simulink library "DF3000_V2_Common"  (R2023b)
settings: Solver=VariableStepAuto  StartTime=0.0  StopTime=10.0  RelTol=1e-3
undefined symbols (not defined in the file): ArmDirSelected, Geom, Newton, Raphson
libraries: simulink_extras x14, $bdroot x7, matrix_library x5, sharedtransform x5, aerolibasang x3, aerolibtransform2 x1
settings Model: Creator=ZJRY  LastModifiedBy=qu_yx

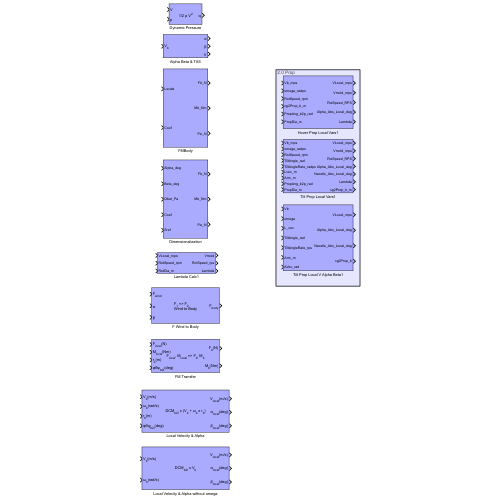
[thumbnail: Simulink's stored preview of the top-level diagram]
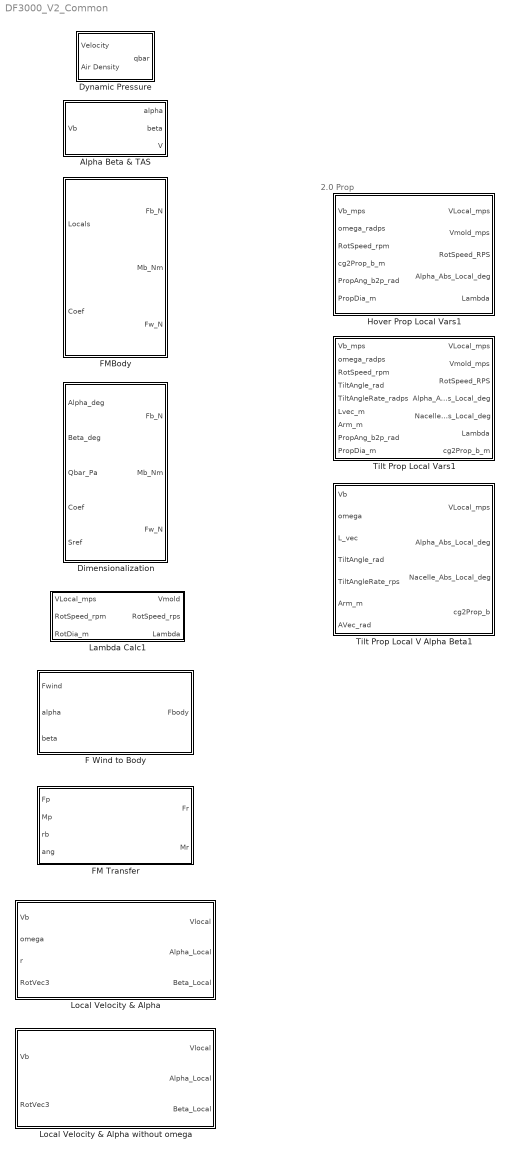
== system DF3000_V2_Common ==
  note: 2.0 Prop
  Alpha Beta & TAS : Subsystem
      mask Display:
      | port_label('input',1,'V_b','texmode','on');
      | port_label('output',1,'\alpha','texmode','on');
      | port_label('output',2,'\beta','texmode','on');
      | port_label('output',3,'V','texmode','on');
  Dimensionalization : Subsystem
  Dynamic Pressure : Subsystem
      mask Display:
      | disp('1/2 \rho V^2', 'texmode','on');
      | port_label('input',1,'V','texmode','on');
      | port_label('input',2,'\rho','texmode','on');
      | port_label('output',1,'q','texmode','on');
  F Wind to Body : Subsystem
      mask Display:
      | disp(['F_1 => F_2 \newline' ...
      |     'Wind to Body'], 'texmode','on');
      | port_label('input',1,'F_{wind}','texmode','on');
      | port_label('input',2,'\alpha','texmode','on');
      | port_label('input',3,'\beta','texmode','on');
      | port_label('output',1,'F_{body}','texmode','on');
  FM Transfer : Subsystem
      mask Display:
      | disp('F_{local}, M_{local} => F_b, M_b', 'texmode','on');
      | port_label('input',1,'F_{local}(N)','texmode','on');
      | port_label('input',2,'M_{local}(Nm)','texmode','on');
      | port_label('input',3,'r_b(m)','texmode','on');
      | port_label('input',4,'\phi\theta\psi_{b2l}(deg)','texmode','on');
      | port_label('output',1,'F_b(N)','texmode','on');
      | port_label('output',2,'M_b(Nm)','texmode','on');
  FMBody : Subsystem
  Hover Prop Local Vars1 : Subsystem
  Lambda Calc1 : Subsystem
  Local Velocity & Alpha : Subsystem
      mask Display:
      | disp('DCM_{b2l} x (V_b + \omega_b x r_b)', 'texmode','on');
      | port_label('input',1,'V_b(m/s)','texmode','on');
      | port_label('input',2,'\omega_b(rad/s)','texmode','on');
      | port_label('input',3,'r_b(m)','texmode','on');
      | port_label('input',4,'\phi\theta\psi_{b2l}(deg)','texmode','on');
      | port_label('output',1,'V_{local}(m/s)','texmode','on');
      | port_label('output',2,'\alpha_{local}(deg)','texmode','on');
      | port_label('output',3,'\beta_{local}(deg)','texmode','on');
  Local Velocity & Alpha without omega : Subsystem
      mask Display:
      | disp('DCM_{b2l} x V_b', 'texmode','on');
      | port_label('input',1,'V_b(m/s)','texmode','on');
      | port_label('input',2,'\omega_b(rad/s)','texmode','on');
      | port_label('output',1,'V_{local}(m/s)','texmode','on');
      | port_label('output',2,'\alpha_{local}(deg)','texmode','on');
      | port_label('output',3,'\beta_{local}(deg)','texmode','on');
  Tilt Prop Local V Alpha Beta1 : Subsystem
  Tilt Prop Local Vars1 : Subsystem

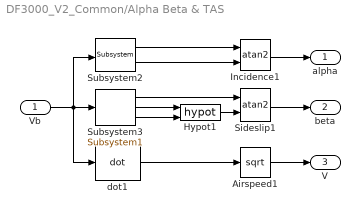
== system DF3000_V2_Common/Alpha Beta & TAS ==
  Vb : Inport
  Airspeed1 : Sqrt  AlgorithmType=Newton-Raphson
  Hypot1 : Math  Operator=hypot
  Incidence1 : Trigonometry  Operator=atan2
  Sideslip1 : Trigonometry  Operator=atan2
  Subsystem2 : aerolibasang/Incidence, Sideslip, & Airspeed/Subsystem  SystemSampleTime=-1  VariantActivationTime=update diagram  AllowFlexibleInterface=on  Latency=0  AutoFrameSizeCalculation=off
  Subsystem3 : aerolibasang/Incidence, Sideslip, & Airspeed/Subsystem1  SystemSampleTime=-1  VariantActivationTime=update diagram  AllowFlexibleInterface=on  Latency=0  AutoFrameSizeCalculation=off
  dot1 : aerolibasang/Incidence, Sideslip, & Airspeed/dot  SystemSampleTime=-1  VariantActivationTime=update diagram  AllowFlexibleInterface=on  Latency=0  AutoFrameSizeCalculation=off
  alpha : Outport
  beta : Outport  Port=2
  V : Outport  Port=3
  wires:
  Vb/1 -> Subsystem3/1, dot1/1, Subsystem2/1
  Subsystem2/2 -> Incidence1/2
  Subsystem3/2 -> Hypot1/1
  Subsystem2/1 -> Incidence1/1
  Subsystem3/3 -> Hypot1/2
  dot1/1 -> Airspeed1/1
  Subsystem3/1 -> Sideslip1/1
  Sideslip1/1 -> beta/1
  Hypot1/1 -> Sideslip1/2
  Airspeed1/1 -> V/1
  Incidence1/1 -> alpha/1

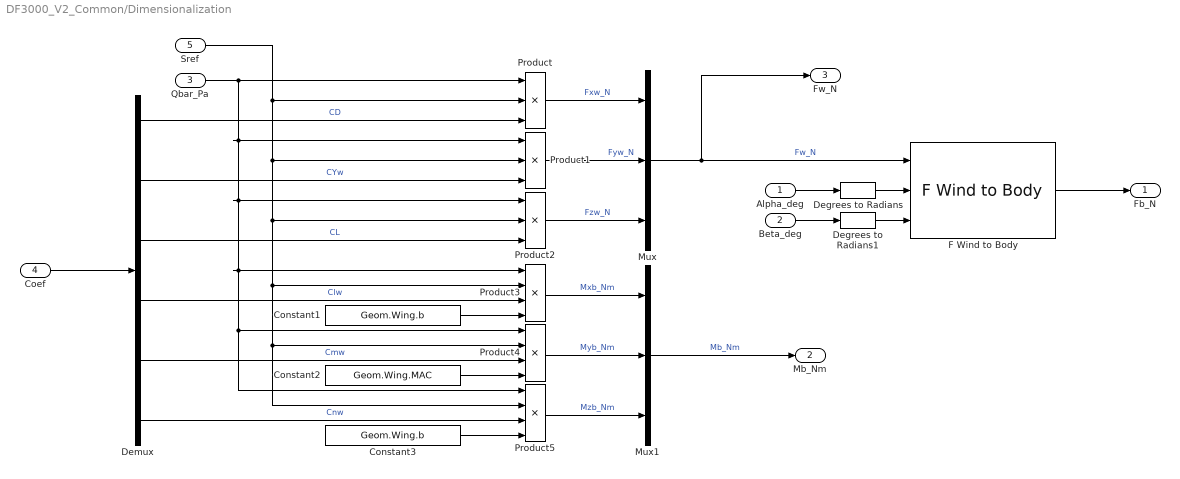
== system DF3000_V2_Common/Dimensionalization ==
  Alpha_deg : Inport
  Beta_deg : Inport  Port=2
  Qbar_Pa : Inport  Port=3
  Coef : Inport  Port=4
  Sref : Inport  Port=5
  Constant1 : Constant  Value=Geom.Wing.b
  Constant2 : Constant  Value=Geom.Wing.MAC
  Constant3 : Constant  Value=Geom.Wing.b
  Degrees to Radians : simulink_extras/Transformations/Degrees to Radians
  Degrees to Radians1 : simulink_extras/Transformations/Degrees to Radians
  Demux : Demux  Outputs=6
  F Wind to Body : $bdroot/F Wind to Body  SystemSampleTime=-1  VariantActivationTime=update diagram  AllowFlexibleInterface=on  Latency=0  AutoFrameSizeCalculation=off
  Mux : Mux  Inputs=3
  Mux1 : Mux  Inputs=3
  Product : Product  Inputs=3
  Product1 : Product  Inputs=3
  Product2 : Product  Inputs=3
  Product3 : Product  Inputs=4
  Product4 : Product  Inputs=4
  Product5 : Product  Inputs=4
  Fb_N : Outport
  Mb_Nm : Outport  Port=2
  Fw_N : Outport  Port=3
  wires:
  Beta_deg/1 -> Degrees to Radians1/1
  Alpha_deg/1 -> Degrees to Radians/1
  F Wind to Body/1 -> Fb_N/1
  Mux1/1 -> Mb_Nm/1  "Mb_Nm"
  Mux/1 -> F Wind to Body/1, Fw_N/1  "Fw_N"
  Constant1/1 -> Product3/4
  Constant3/1 -> Product5/4
  Constant2/1 -> Product4/4
  Sref/1 -> Product5/2, Product4/2, Product3/2, Product2/2, Product1/2, Product/2
  Demux/6 -> Product5/3  "Cnw"
  Demux/5 -> Product4/3  "Cmw"
  Demux/4 -> Product3/3  "Clw"
  Product3/1 -> Mux1/1  "Mxb_Nm"
  Product4/1 -> Mux1/2  "Myb_Nm"
  Product5/1 -> Mux1/3  "Mzb_Nm"
  Product2/1 -> Mux/3  "Fzw_N"
  Product1/1 -> Mux/2  "Fyw_N"
  Product/1 -> Mux/1  "Fxw_N"
  Qbar_Pa/1 -> Product1/1, Product2/1, Product4/1, Product5/1, Product3/1, Product/1
  Demux/3 -> Product2/3  "CL"
  Demux/2 -> Product1/3  "CYw"
  Demux/1 -> Product/3  "CD"
  Coef/1 -> Demux/1
  Degrees to Radians/1 -> F Wind to Body/2
  Degrees to Radians1/1 -> F Wind to Body/3

== system DF3000_V2_Common/Dynamic Pressure ==
  Velocity : Inport
  Air Density : Inport  Port=2
  1/2rhoV^2 : Gain  Gain=1/2  SaturateOnIntegerOverflow=on  OutDataTypeStr=Inherit: Same as input  ParamDataTypeStr=Inherit: Same as input
  Add : Sum  Inputs=+++
  Demux1 : Demux  Outputs=3
  Product2 : Product  InputSameDT=on  SaturateOnIntegerOverflow=on  OutDataTypeStr=Inherit: Same as first input
  Square : Math  Operator=square
  Square1 : Math  Operator=square
  Square2 : Math  Operator=square
  qbar : Outport  InitialOutput=0  VectorParamsAs1DForOutWhenUnconnected=off
  wires:
  Air Density/1 -> Product2/2
  Product2/1 -> 1/2rhoV^2/1
  1/2rhoV^2/1 -> qbar/1
  Add/1 -> Product2/1
  Demux1/3 -> Square/1
  Velocity/1 -> Demux1/1
  Square/1 -> Add/3
  Demux1/1 -> Square2/1
  Demux1/2 -> Square1/1
  Square1/1 -> Add/2
  Square2/1 -> Add/1

== system DF3000_V2_Common/F Wind to Body ==
  Fwind : Inport  PortDimensions=3
  alpha : Inport  Port=2
  beta : Inport  Port=3
  Direction Cosine Matrix Body to Wind : aerolibtransform2/Direction Cosine Matrix Body to Wind
  Matrix Multiply3 : Product  Multiplication=Matrix(*)
  Mux : Mux  Inputs=2
  Wind to Body : Math  Operator=transpose
  Fbody : Outport  PortDimensions=3
  wires:
  Matrix Multiply3/1 -> Fbody/1
  Direction Cosine Matrix Body to Wind/1 -> Wind to Body/1
  Fwind/1 -> Matrix Multiply3/2
  Mux/1 -> Direction Cosine Matrix Body to Wind/1
  alpha/1 -> Mux/1
  beta/1 -> Mux/2
  Wind to Body/1 -> Matrix Multiply3/1

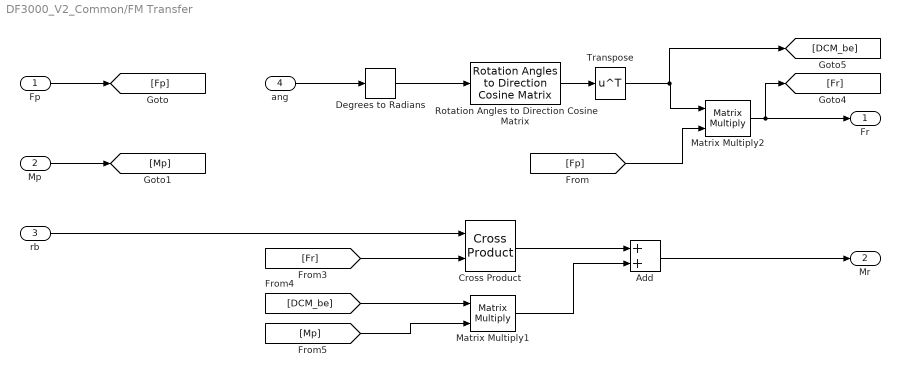
== system DF3000_V2_Common/FM Transfer ==
  Fp : Inport  PortDimensions=3
  Mp : Inport  Port=2  PortDimensions=3
  rb : Inport  Port=3  PortDimensions=3
  ang : Inport  Port=4  PortDimensions=3
  Add : Sum
  Cross Product : matrix_library/Cross Product
  Degrees to Radians : simulink_extras/Transformations/Degrees to Radians
  Matrix Multiply1 : Product  Multiplication=Matrix(*)
  Matrix Multiply2 : Product  Multiplication=Matrix(*)
  Rotation Angles to Direction Cosine Matrix : sharedtransform/Rotation Angles to Direction Cosine Matrix  rotationOrder=XYZ  aMode=aMode
  Transpose : Math  Operator=transpose
  Fr : Outport  PortDimensions=3
  Mr : Outport  Port=2  PortDimensions=3
  wires:
  rb/1 -> Cross Product/1
  [Fp] -> Matrix Multiply2/2
  Rotation Angles to Direction Cosine Matrix/1 -> Transpose/1
  Degrees to Radians/1 -> Rotation Angles to Direction Cosine Matrix/1
  Fp/1 -> [Fp]
  Transpose/1 -> Matrix Multiply2/1, [DCM_be]
  Mp/1 -> [Mp]
  Add/1 -> Mr/1
  ang/1 -> Degrees to Radians/1
  Matrix Multiply2/1 -> Fr/1, [Fr]
  [DCM_be] -> Matrix Multiply1/1
  [Fr] -> Cross Product/2
  Cross Product/1 -> Add/1
  [Mp] -> Matrix Multiply1/2
  Matrix Multiply1/1 -> Add/2

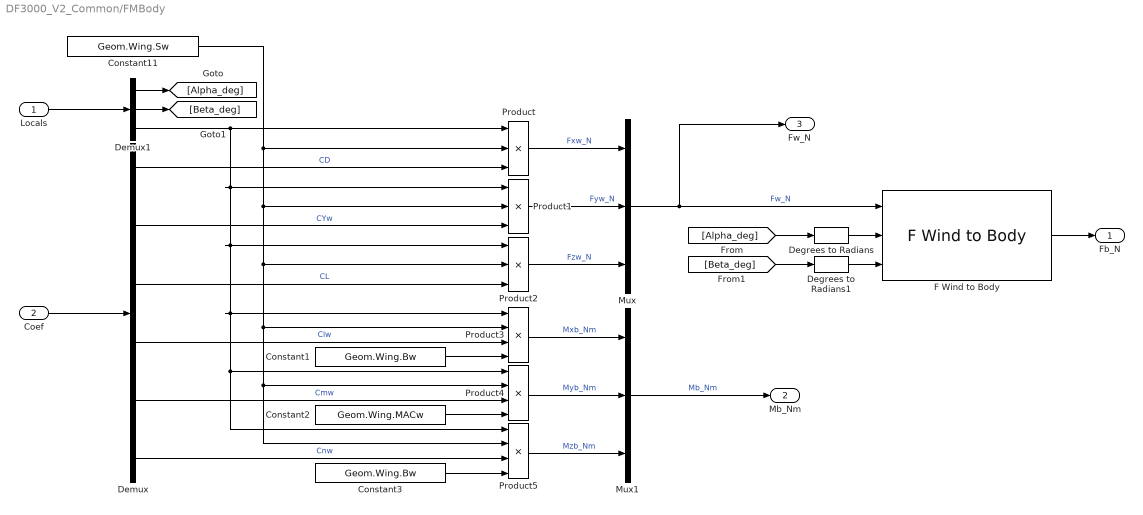
== system DF3000_V2_Common/FMBody ==
  Locals : Inport
  Coef : Inport  Port=2
  Constant1 : Constant  Value=Geom.Wing.Bw
  Constant11 : Constant  Value=Geom.Wing.Sw
  Constant2 : Constant  Value=Geom.Wing.MACw
  Constant3 : Constant  Value=Geom.Wing.Bw
  Degrees to Radians : simulink_extras/Transformations/Degrees to Radians
  Degrees to Radians1 : simulink_extras/Transformations/Degrees to Radians
  Demux : Demux  Outputs=6
  Demux1 : Demux  Outputs=3
  F Wind to Body : $bdroot/F Wind to Body  SystemSampleTime=-1  VariantActivationTime=update diagram  AllowFlexibleInterface=on  Latency=0  AutoFrameSizeCalculation=off
  Mux : Mux  Inputs=3
  Mux1 : Mux  Inputs=3
  Product : Product  Inputs=3
  Product1 : Product  Inputs=3
  Product2 : Product  Inputs=3
  Product3 : Product  Inputs=4
  Product4 : Product  Inputs=4
  Product5 : Product  Inputs=4
  Fb_N : Outport
  Mb_Nm : Outport  Port=2
  Fw_N : Outport  Port=3
  wires:
  [Beta_deg] -> Degrees to Radians1/1
  [Alpha_deg] -> Degrees to Radians/1
  Demux1/1 -> [Alpha_deg]
  F Wind to Body/1 -> Fb_N/1
  Mux1/1 -> Mb_Nm/1  "Mb_Nm"
  Mux/1 -> F Wind to Body/1, Fw_N/1  "Fw_N"
  Constant1/1 -> Product3/4
  Constant3/1 -> Product5/4
  Constant2/1 -> Product4/4
  Constant11/1 -> Product5/2, Product4/2, Product3/2, Product2/2, Product1/2, Product/2
  Demux/6 -> Product5/3  "Cnw"
  Demux/5 -> Product4/3  "Cmw"
  Demux/4 -> Product3/3  "Clw"
  Product3/1 -> Mux1/1  "Mxb_Nm"
  Product4/1 -> Mux1/2  "Myb_Nm"
  Product5/1 -> Mux1/3  "Mzb_Nm"
  Product2/1 -> Mux/3  "Fzw_N"
  Product1/1 -> Mux/2  "Fyw_N"
  Product/1 -> Mux/1  "Fxw_N"
  Demux1/3 -> Product1/1, Product2/1, Product4/1, Product5/1, Product3/1, Product/1
  Locals/1 -> Demux1/1
  Demux/3 -> Product2/3  "CL"
  Demux/2 -> Product1/3  "CYw"
  Demux/1 -> Product/3  "CD"
  Coef/1 -> Demux/1
  Degrees to Radians/1 -> F Wind to Body/2
  Degrees to Radians1/1 -> F Wind to Body/3
  Demux1/2 -> [Beta_deg]

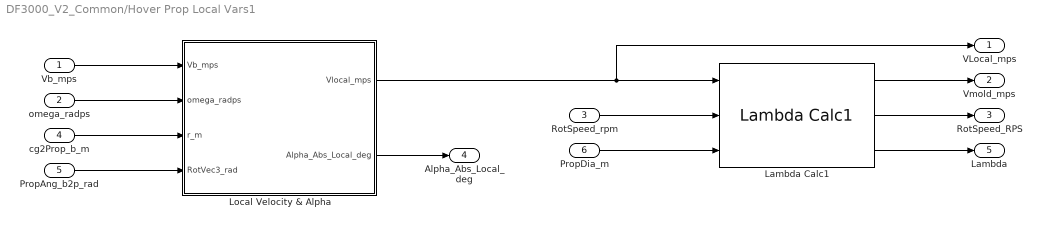
== system DF3000_V2_Common/Hover Prop Local Vars1 ==
  Vb_mps : Inport
  omega_radps : Inport  Port=2
  RotSpeed_rpm : Inport  Port=3
  cg2Prop_b_m : Inport  Port=4
  PropAng_b2p_rad : Inport  Port=5
  PropDia_m : Inport  Port=6
  Lambda Calc1 : $bdroot/Lambda Calc1  SystemSampleTime=-1  VariantActivationTime=update diagram  AllowFlexibleInterface=on  Latency=0  AutoFrameSizeCalculation=off
  Local Velocity & Alpha : Subsystem
  VLocal_mps : Outport
  Vmold_mps : Outport  Port=2
  RotSpeed_RPS : Outport  Port=3
  Alpha_Abs_Local_deg : Outport  Port=4
  Lambda : Outport  Port=5
  wires:
  omega_radps/1 -> Local Velocity & Alpha/2(omega_radps)
  RotSpeed_rpm/1 -> Lambda Calc1/2
  Local Velocity & Alpha/1(Vlocal_mps) -> Lambda Calc1/1, VLocal_mps/1
  Vb_mps/1 -> Local Velocity & Alpha/1(Vb_mps)
  Local Velocity & Alpha/2(Alpha_Abs_Local_deg) -> Alpha_Abs_Local_deg/1
  PropAng_b2p_rad/1 -> Local Velocity & Alpha/4(RotVec3_rad)
  cg2Prop_b_m/1 -> Local Velocity & Alpha/3(r_m)
  PropDia_m/1 -> Lambda Calc1/3
  Lambda Calc1/3 -> Lambda/1
  Lambda Calc1/2 -> RotSpeed_RPS/1
  Lambda Calc1/1 -> Vmold_mps/1

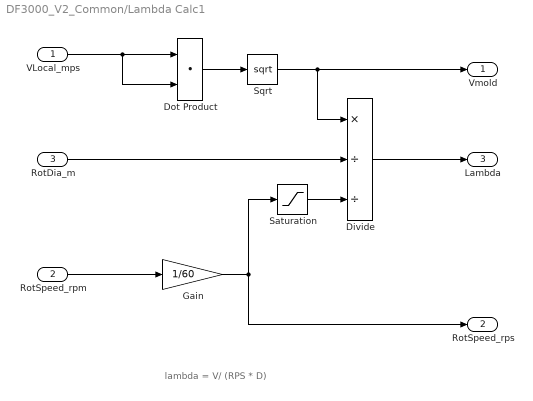
== system DF3000_V2_Common/Lambda Calc1 ==
  note: lambda = V/ (RPS * D)
  VLocal_mps : Inport
  RotSpeed_rpm : Inport  Port=2
  RotDia_m : Inport  Port=3
  Divide : Product  Inputs=*//
  Dot Product : DotProduct  OutDataTypeStr=Inherit: Inherit via internal rule
  Gain : Gain  Gain=1/60
  Saturation : Saturate  UpperLimit=10000  LowerLimit=0.0001
  Sqrt : Sqrt
  Vmold : Outport
  RotSpeed_rps : Outport  Port=2
  Lambda : Outport  Port=3
  wires:
  RotSpeed_rpm/1 -> Gain/1
  Gain/1 -> Saturation/1, RotSpeed_rps/1
  RotDia_m/1 -> Divide/2
  Divide/1 -> Lambda/1
  VLocal_mps/1 -> Dot Product/2, Dot Product/1
  Dot Product/1 -> Sqrt/1
  Saturation/1 -> Divide/3
  Sqrt/1 -> Vmold/1, Divide/1

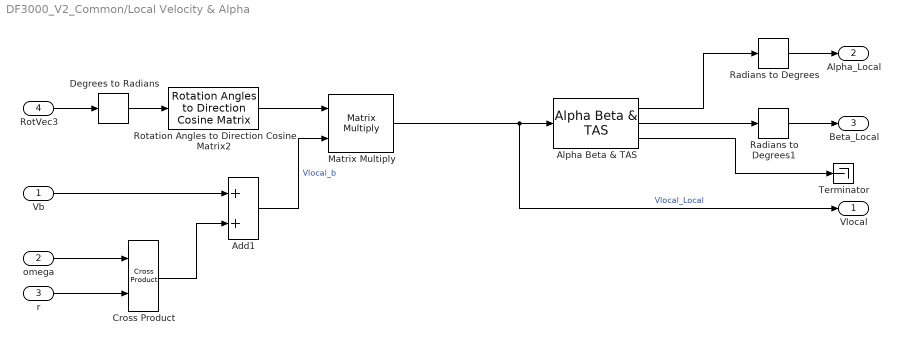
== system DF3000_V2_Common/Local Velocity & Alpha ==
  Vb : Inport
  omega : Inport  Port=2
  r : Inport  Port=3
  RotVec3 : Inport  Port=4
  Add1 : Sum
  Alpha Beta & TAS : $bdroot/Alpha Beta & TAS  SystemSampleTime=-1  VariantActivationTime=update diagram  AllowFlexibleInterface=on  Latency=0  AutoFrameSizeCalculation=off
  Cross Product : matrix_library/Cross Product
  Degrees to Radians : simulink_extras/Transformations/Degrees to Radians
  Matrix Multiply : Product  Multiplication=Matrix(*)
  Radians to Degrees : simulink_extras/Transformations/Radians to Degrees
  Radians to Degrees1 : simulink_extras/Transformations/Radians to Degrees
  Rotation Angles to Direction Cosine Matrix2 : sharedtransform/Rotation Angles to Direction Cosine Matrix  rotationOrder=XYZ  aMode=aMode
  Terminator : Terminator
  Vlocal : Outport
  Alpha_Local : Outport  Port=2
  Beta_Local : Outport  Port=3
  wires:
  Vb/1 -> Add1/1
  Add1/1 -> Matrix Multiply/2  "Vlocal_b"
  Cross Product/1 -> Add1/2
  r/1 -> Cross Product/2
  omega/1 -> Cross Product/1
  Matrix Multiply/1 -> Vlocal/1, Alpha Beta & TAS/1  "Vlocal_Local"
  Rotation Angles to Direction Cosine Matrix2/1 -> Matrix Multiply/1
  RotVec3/1 -> Degrees to Radians/1
  Alpha Beta & TAS/3 -> Terminator/1
  Degrees to Radians/1 -> Rotation Angles to Direction Cosine Matrix2/1
  Alpha Beta & TAS/1 -> Radians to Degrees/1
  Alpha Beta & TAS/2 -> Radians to Degrees1/1
  Radians to Degrees/1 -> Alpha_Local/1
  Radians to Degrees1/1 -> Beta_Local/1

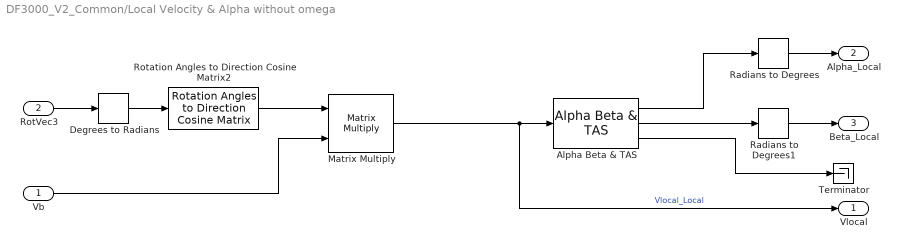
== system DF3000_V2_Common/Local Velocity & Alpha without omega ==
  Vb : Inport
  RotVec3 : Inport  Port=2
  Alpha Beta & TAS : $bdroot/Alpha Beta & TAS  SystemSampleTime=-1  VariantActivationTime=update diagram  AllowFlexibleInterface=on  Latency=0  AutoFrameSizeCalculation=off
  Degrees to Radians : simulink_extras/Transformations/Degrees to Radians
  Matrix Multiply : Product  Multiplication=Matrix(*)
  Radians to Degrees : simulink_extras/Transformations/Radians to Degrees
  Radians to Degrees1 : simulink_extras/Transformations/Radians to Degrees
  Rotation Angles to Direction Cosine Matrix2 : sharedtransform/Rotation Angles to Direction Cosine Matrix  rotationOrder=XYZ  aMode=aMode
  Terminator : Terminator
  Vlocal : Outport
  Alpha_Local : Outport  Port=2
  Beta_Local : Outport  Port=3
  wires:
  Radians to Degrees1/1 -> Beta_Local/1
  Radians to Degrees/1 -> Alpha_Local/1
  Alpha Beta & TAS/2 -> Radians to Degrees1/1
  Alpha Beta & TAS/1 -> Radians to Degrees/1
  Degrees to Radians/1 -> Rotation Angles to Direction Cosine Matrix2/1
  Alpha Beta & TAS/3 -> Terminator/1
  RotVec3/1 -> Degrees to Radians/1
  Rotation Angles to Direction Cosine Matrix2/1 -> Matrix Multiply/1
  Matrix Multiply/1 -> Alpha Beta & TAS/1, Vlocal/1  "Vlocal_Local"
  Vb/1 -> Matrix Multiply/2

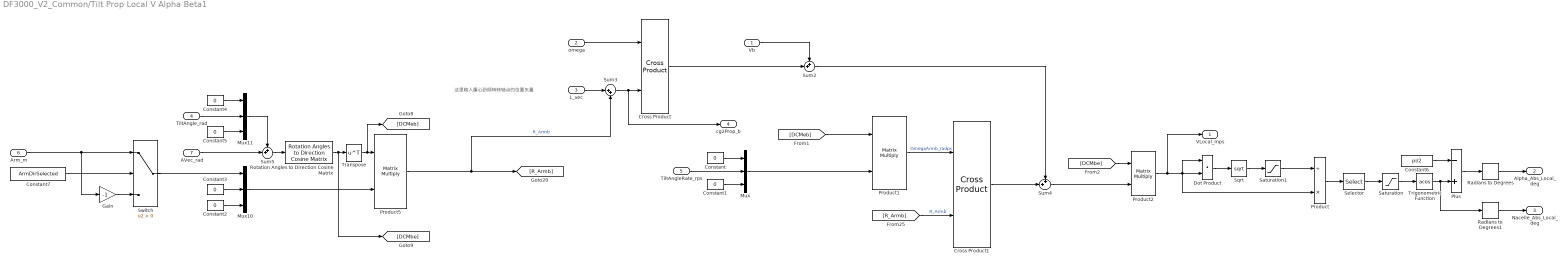
== system DF3000_V2_Common/Tilt Prop Local V Alpha Beta1 ==
  note: 这里输入重心到倾转转轴点的位置矢量
  Vb : Inport
  omega : Inport  Port=2
  L_vec : Inport  Port=3
  TiltAngle_rad : Inport  Port=4
  TiltAngleRate_rps : Inport  Port=5
  Arm_m : Inport  Port=6
  AVec_rad : Inport  Port=7
  Constant{,1..5} (6 alike) : Constant  Value=0
  Constant6 : Constant  Value=pi/2
  Constant7 : Constant  Value=ArmDirSelected
  Cross Product : matrix_library/Cross Product
  Cross Product1 : matrix_library/Cross Product
  Dot Product : DotProduct  OutDataTypeStr=Inherit: Inherit via internal rule
  Gain : Gain  Gain=-1
  Mux : Mux  Inputs=3
  Mux10 : Mux  Inputs=3
  Mux11 : Mux  Inputs=3
  Plus : Sum  Inputs=-+
  Product : Product  Inputs=/*
  Product1 : Product  Multiplication=Matrix(*)  InputSameDT=on  SaturateOnIntegerOverflow=on  OutDataTypeStr=Inherit: Same as first input
  Product2 : Product  Multiplication=Matrix(*)  InputSameDT=on  SaturateOnIntegerOverflow=on  OutDataTypeStr=Inherit: Same as first input
  Product5 : Product  Multiplication=Matrix(*)  InputSameDT=on  SaturateOnIntegerOverflow=on  OutDataTypeStr=Inherit: Same as first input
  Radians to Degrees : simulink_extras/Transformations/Radians to Degrees
  Radians to Degrees1 : simulink_extras/Transformations/Radians to Degrees
  Rotation Angles to Direction Cosine Matrix : sharedtransform/Rotation Angles to Direction Cosine Matrix  rotationOrder=XYZ  aMode=aMode
  Saturation : Saturate  UpperLimit=1  LowerLimit=-1
  Saturation1 : Saturate  UpperLimit=inf  LowerLimit=0.0001
  Selector : Selector  InputPortWidth=3  IndexOptions=Index vector (dialog)  Indices=[1]  OutputSizes=1
  Sqrt : Sqrt
  Sum2 : Sum  Inputs=++|
  Sum3 : Sum  Inputs=|++
  Sum4 : Sum  Inputs=++|
  Sum5 : Sum  Inputs=++|
  Switch : Switch  Criteria=u2 > Threshold  SaturateOnIntegerOverflow=off  InputSameDT=off
  Transpose : Math  Operator=transpose
  Trigonometric Function : Trigonometry  Operator=acos
  VLocal_mps : Outport
  Alpha_Abs_Local_deg : Outport  Port=2
  Nacelle_Abs_Local_deg : Outport  Port=3
  cg2Prop_b : Outport  Port=4
  wires:
  Constant5/1 -> Mux11/3
  Cross Product1/1 -> Sum4/2
  [R_Armb] -> Cross Product1/2  "R_Armb"
  TiltAngleRate_rps/1 -> Mux/2
  Product1/1 -> Cross Product1/1  "OmegaArmb_radps"
  [DCMeb] -> Product1/1
  Transpose/1 -> [DCMeb], Product5/1
  [DCMbe] -> Product2/1
  Sum3/1 -> cg2Prop_b/1, Cross Product/2
  Constant/1 -> Mux/1
  Product5/1 -> [R_Armb], Sum3/2  "R_Armb"
  Constant1/1 -> Mux/3
  Rotation Angles to Direction Cosine Matrix/1 -> [DCMbe], Transpose/1
  omega/1 -> Cross Product/1
  TiltAngle_rad/1 -> Mux11/2
  Cross Product/1 -> Sum2/2
  Mux10/1 -> Product5/2
  Sum2/1 -> Sum4/1
  AVec_rad/1 -> Sum5/2
  Sum4/1 -> Product2/2
  Sum5/1 -> Rotation Angles to Direction Cosine Matrix/1
  Constant4/1 -> Mux11/1
  Mux11/1 -> Sum5/1
  Mux/1 -> Product1/2
  Constant3/1 -> Mux10/2
  Constant2/1 -> Mux10/3
  Arm_m/1 -> Switch/1, Gain/1
  Gain/1 -> Switch/3
  Constant7/1 -> Switch/2
  Switch/1 -> Mux10/1
  Constant6/1 -> Plus/1
  Selector/1 -> Saturation/1
  Trigonometric Function/1 -> Radians to Degrees1/1, Plus/2
  Product/1 -> Selector/1
  Plus/1 -> Radians to Degrees/1
  Radians to Degrees/1 -> Alpha_Abs_Local_deg/1
  Product2/1 -> Product/2, Dot Product/1, Dot Product/2, VLocal_mps/1
  Dot Product/1 -> Sqrt/1
  Saturation/1 -> Trigonometric Function/1
  Sqrt/1 -> Saturation1/1
  L_vec/1 -> Sum3/1
  Vb/1 -> Sum2/1
  Radians to Degrees1/1 -> Nacelle_Abs_Local_deg/1
  Saturation1/1 -> Product/1

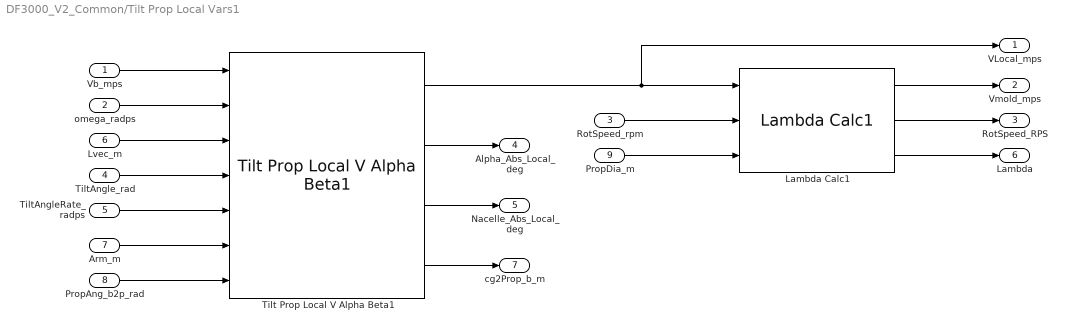
== system DF3000_V2_Common/Tilt Prop Local Vars1 ==
  Vb_mps : Inport
  omega_radps : Inport  Port=2
  RotSpeed_rpm : Inport  Port=3
  TiltAngle_rad : Inport  Port=4
  TiltAngleRate_radps : Inport  Port=5
  Lvec_m : Inport  Port=6
  Arm_m : Inport  Port=7
  PropAng_b2p_rad : Inport  Port=8
  PropDia_m : Inport  Port=9
  Lambda Calc1 : $bdroot/Lambda Calc1  SystemSampleTime=-1  VariantActivationTime=update diagram  AllowFlexibleInterface=on  Latency=0  AutoFrameSizeCalculation=off
  Tilt Prop Local V Alpha Beta1 : $bdroot/Tilt Prop Local V Alpha Beta1  SystemSampleTime=-1  VariantActivationTime=update diagram  AllowFlexibleInterface=on  Latency=0  AutoFrameSizeCalculation=off
  VLocal_mps : Outport
  Vmold_mps : Outport  Port=2
  RotSpeed_RPS : Outport  Port=3
  Alpha_Abs_Local_deg : Outport  Port=4
  Nacelle_Abs_Local_deg : Outport  Port=5
  Lambda : Outport  Port=6
  cg2Prop_b_m : Outport  Port=7
  wires:
  Tilt Prop Local V Alpha Beta1/4 -> cg2Prop_b_m/1
  Tilt Prop Local V Alpha Beta1/3 -> Nacelle_Abs_Local_deg/1
  Lambda Calc1/1 -> Vmold_mps/1
  Lambda Calc1/2 -> RotSpeed_RPS/1
  Lambda Calc1/3 -> Lambda/1
  Tilt Prop Local V Alpha Beta1/2 -> Alpha_Abs_Local_deg/1
  Vb_mps/1 -> Tilt Prop Local V Alpha Beta1/1
  Tilt Prop Local V Alpha Beta1/1 -> Lambda Calc1/1, VLocal_mps/1
  PropDia_m/1 -> Lambda Calc1/3
  RotSpeed_rpm/1 -> Lambda Calc1/2
  omega_radps/1 -> Tilt Prop Local V Alpha Beta1/2
  Arm_m/1 -> Tilt Prop Local V Alpha Beta1/6
  PropAng_b2p_rad/1 -> Tilt Prop Local V Alpha Beta1/7
  TiltAngle_rad/1 -> Tilt Prop Local V Alpha Beta1/4
  TiltAngleRate_radps/1 -> Tilt Prop Local V Alpha Beta1/5
  Lvec_m/1 -> Tilt Prop Local V Alpha Beta1/3

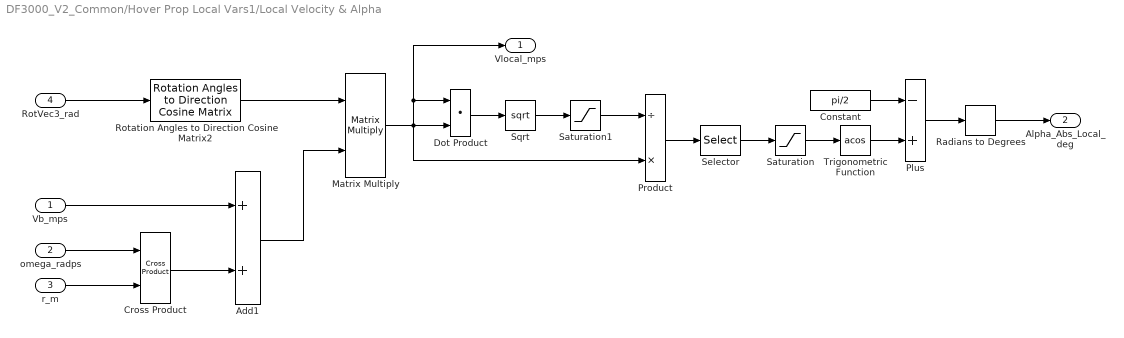
== system DF3000_V2_Common/Hover Prop Local Vars1/Local Velocity & Alpha ==
  Vb_mps : Inport
  omega_radps : Inport  Port=2
  r_m : Inport  Port=3
  RotVec3_rad : Inport  Port=4
  Add1 : Sum
  Constant : Constant  Value=pi/2
  Cross Product : matrix_library/Cross Product
  Dot Product : DotProduct  OutDataTypeStr=Inherit: Inherit via internal rule
  Matrix Multiply : Product  Multiplication=Matrix(*)
  Plus : Sum  Inputs=-+
  Product : Product  Inputs=/*
  Radians to Degrees : simulink_extras/Transformations/Radians to Degrees
  Rotation Angles to Direction Cosine Matrix2 : sharedtransform/Rotation Angles to Direction Cosine Matrix  rotationOrder=XYZ  aMode=aMode
  Saturation : Saturate  UpperLimit=1  LowerLimit=-1
  Saturation1 : Saturate  UpperLimit=inf  LowerLimit=0.0001
  Selector : Selector  InputPortWidth=3  IndexOptions=Index vector (dialog)  Indices=[1]  OutputSizes=1
  Sqrt : Sqrt
  Trigonometric Function : Trigonometry  Operator=acos
  Vlocal_mps : Outport
  Alpha_Abs_Local_deg : Outport  Port=2
  wires:
  Saturation1/1 -> Product/1
  Plus/1 -> Radians to Degrees/1
  Constant/1 -> Plus/1
  Trigonometric Function/1 -> Plus/2
  Radians to Degrees/1 -> Alpha_Abs_Local_deg/1
  Saturation/1 -> Trigonometric Function/1
  Selector/1 -> Saturation/1
  Product/1 -> Selector/1
  Sqrt/1 -> Saturation1/1
  Dot Product/1 -> Sqrt/1
  Vb_mps/1 -> Add1/1
  Add1/1 -> Matrix Multiply/2
  Cross Product/1 -> Add1/2
  r_m/1 -> Cross Product/2
  omega_radps/1 -> Cross Product/1
  Matrix Multiply/1 -> Dot Product/2, Dot Product/1, Vlocal_mps/1, Product/2
  Rotation Angles to Direction Cosine Matrix2/1 -> Matrix Multiply/1
  RotVec3_rad/1 -> Rotation Angles to Direction Cosine Matrix2/1
